simulink model "DatosIdent"  (R2022b)
settings: Solver=VariableStepAuto  StartTime=0.0  StopTime=10.0  RelTol=1e-3
undefined symbols (not defined in the file): sigbuilder_block
libraries: arduinolib x1
settings Model: Creator=Usuario  LastModifiedBy=dar.io

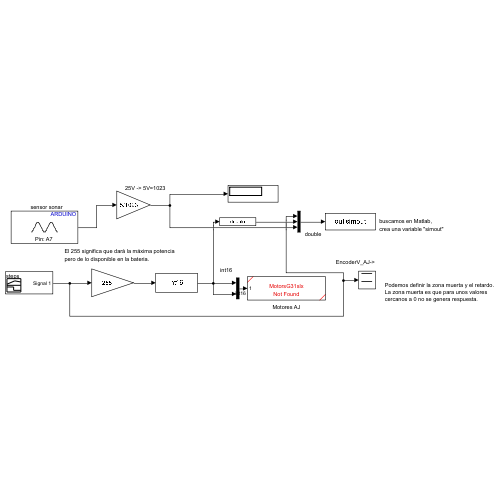
[thumbnail: Simulink's stored preview of the top-level diagram]
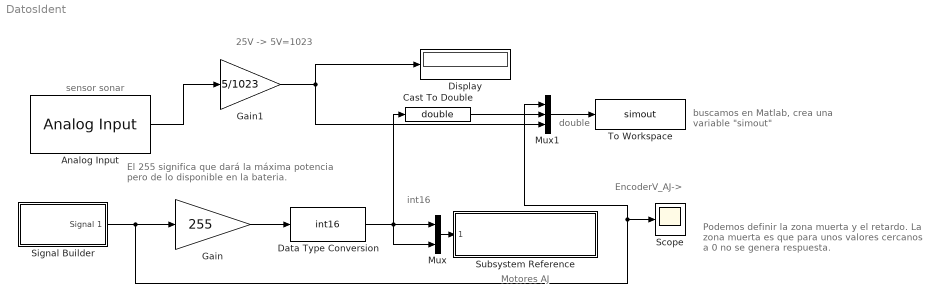
== system DatosIdent ==
  note: sensor sonar
  note: 25V -> 5V=1023
  note: El 255 significa que dará la máxima potencia
      | pero de lo disponible en la bateria.
  note: Podemos definir la zona muerta y el retardo.
      | La zona muerta es que para unos valores
      | cercanos a 0 no se genera respuesta.
  note: buscamos en Matlab,
      | crea una variable "simout"
  note: int16
  note: double
  note: EncoderV_AJ->
  note: Motores AJ
  Analog Input : arduinolib/Analog Input  pinNumber=7  ReadResultsOnly=off  ConversionTriggerSource=Software  ExternalTriggerType=uint32( 0 )  OutputDataType=uint16  EnableConversionCompleteNotify=off  EnableOuputStatus=off  SampleTime=-1  blockPlatform=arduino
  Cast To Double : DataTypeConversion  OutDataTypeStr=double  SaturateOnIntegerOverflow=off  RndMeth=Floor
  Data Type Conversion : DataTypeConversion  OutDataTypeStr=int16  SaturateOnIntegerOverflow=off  RndMeth=Floor
  Display : Display
  Gain : Gain  Gain=255
  Gain1 : Gain  Gain=5/1023
  Mux : Mux  Inputs=2
  Mux1 : Mux  Inputs=3
  Scope : Scope
  Signal Builder : Subsystem  Tag=STV Subsys  LoadFcn=sigbuilder_block('load');  StartFcn=sigbuilder_block('start');  StopFcn=sigbuilder_block('stop');  ClipboardFcn=sigbuilder_block('clipboard');  mask(Sigbuilder block){tuvar=[0:10]}
      mask help: Simulink:masks:SigbuilderBlock_MD
      mask init:
      | if ~strcmp(get_param(bdroot(gcbh),'SimulationStatus'),'stopped') tuvar = sigbuilder_block('maskInit'); end
      settings: CopyFcn=sigbuilder_block('copy');  DeleteFcn=sigbuilder_block('delete');  ModelCloseFcn=sigbuilder_block('modelClose');  PreSaveFcn=sigbuilder_block('preSave');  PauseFcn=sigbuilder_block('pause');  ContinueFcn=sigbuilder_block('continue');  NameChangeFcn=sigbuilder_block('namechange');  OpenFcn=sigbuilder_block('open',[200.4 104.4 528 400.2 ]);  CloseFcn=sigbuilder_block('close');
      mask Display: plot(0, 0, 100, 100,[2, 2, 32, 32, 2], [68, 8, 8, 68, 68],[32, 2], [38, 38], [32, 19, 2],[53, 60, 44], [32, 17, 17, 2],[16, 16, 31, 31]);txt = getActiveGroup(gcbh);text(2, 100, txt,'verticalAlignment', 'top');
  Subsystem Reference : Subsystem  ReferencedSubsystem=MotorsG31slx
  To Workspace : ToWorkspace  VariableName=simout  SaveFormat=Timeseries  SampleTime=-1
  wires:
  Signal Builder/1(Signal 1) -> Scope/1, Mux1/1, Gain/1
  Mux1/1 -> To Workspace/1
  Data Type Conversion/1 -> Cast To Double/1, Mux/1, Mux/2
  Gain/1 -> Data Type Conversion/1
  Analog Input/1 -> Gain1/1
  Gain1/1 -> Display/1, Mux1/3
  Cast To Double/1 -> Mux1/2
  Mux/1 -> Subsystem Reference/1

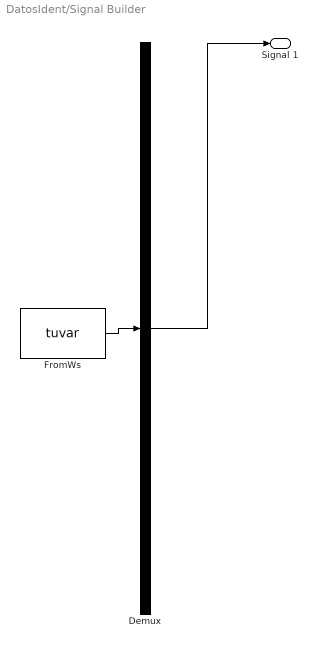
== system DatosIdent/Signal Builder ==
  Demux : Demux  Tag=STV Demux  Outputs=1
      settings: DisplayOption=none
  FromWs : FromWorkspace  Tag=STV FromWs  VariableName=tuvar
      SigBuilderData=|
      | common.afterFinalStr = 'Extrapolate'
      | common.sampleTime = 0
      | dataSet(1).timeRange = [0 10]
      | dataSet(1).name = 'rampa'
      | dataSet(2).timeRange = [0 10]
      | dataSet(2).name = 'steps'
      | sbobj.Groups(1).Name = 'rampa'
      | sbobj.Groups(1).Signals.Name = 'Signal 1'
      | sbobj.Groups(1).Signals.XData = [0 2.5 7.5 10]
      | sbobj.Groups(1).Signals.YData = [0 1 -1 0]
      | sbobj.Groups(2).Name = 'steps'
      | sbobj.Groups(2).Signals.Name = 'Signal 1'
      | sbobj.Groups(2).Signals.XData = [0 1 1 2.5 2.5 4 4 5.5 5.5 7 7 8.5 8.5 10]
      | sbobj.Groups(2).Signals.YData = [0 0 1 1 -1 -1 1 1 -0.99 -1 1 1 0 0]
  Signal 1 : Outport  Tag=STV Outport
  wires:
  Demux/1 -> Signal 1/1
  FromWs/1 -> Demux/1
